simulink model "Sim1_3_simu"  (R2021a)
settings: Solver=VariableStepAuto  StartTime=0.0  StopTime=Ts*1e6  RelTol=1e-3
values from neighbouring files (symbols this model uses):
  sysd = c2d(G, Ts, 'zoh')    [Sim1_1.m]    (also in Sim1_2.m; Sim1_2_5.m; Sim1_2_CovRes_Fast.m; Sim1_2_CovRes_Slow.m)
  Ts = (2*pi)/(20*bw)    [Sim1_1.m]    (also in Sim1_2.m; Sim1_2_5.m; Sim1_2_CovRes_Fast.m; Sim1_2_CovRes_Slow.m)
undefined symbols (not defined in the file or in its folder): C
settings Model: Creator=ASUS  LastModifiedBy=ASUS

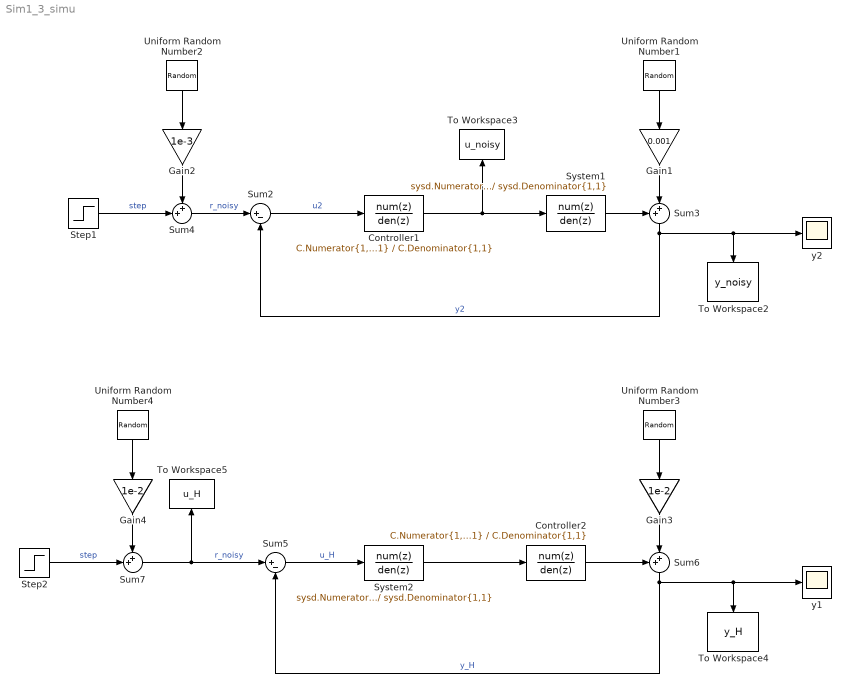
== system Sim1_3_simu ==
  Controller1 : DiscreteTransferFcn  Numerator=C.Numerator{1,1}  Denominator=C.Denominator{1,1}
  Controller2 : DiscreteTransferFcn  Numerator=C.Numerator{1,1}  Denominator=C.Denominator{1,1}
  Gain1 : Gain  Gain=0.001
  Gain2 : Gain  Gain=1e-3
  Gain3 : Gain  Gain=1e-2
  Gain4 : Gain  Gain=1e-2
  Step1 : Step  Time=0  SampleTime=0
  Step2 : Step  Time=0  SampleTime=0
  Sum2 : Sum  Inputs=|+-
  Sum{3..4,6..7} (4 alike) : Sum  Inputs=++|
  Sum5 : Sum  Inputs=|+-
  System1 : DiscreteTransferFcn  Numerator=sysd.Numerator{1,1}  Denominator=sysd.Denominator{1,1}
  System2 : DiscreteTransferFcn  Numerator=sysd.Numerator{1,1}  Denominator=sysd.Denominator{1,1}
  To Workspace2 : ToWorkspace  VariableName=y_noisy  SampleTime=-1
  To Workspace3 : ToWorkspace  VariableName=u_noisy  SampleTime=-1
  To Workspace4 : ToWorkspace  VariableName=y_H  SampleTime=-1
  To Workspace5 : ToWorkspace  VariableName=u_H  SampleTime=-1
  Uniform Random Number1 : UniformRandomNumber  SampleTime=Ts
  Uniform Random Number2 : UniformRandomNumber  Seed=1  SampleTime=Ts
  Uniform Random Number3 : UniformRandomNumber  SampleTime=Ts
  Uniform Random Number4 : UniformRandomNumber  Seed=1  SampleTime=Ts
  y1 : Scope
  y2 : Scope
  wires:
  Sum3/1 -> Sum2/2, y2/1, To Workspace2/1  "y2"
  Gain1/1 -> Sum3/2
  Uniform Random Number1/1 -> Gain1/1
  Uniform Random Number2/1 -> Gain2/1
  Gain2/1 -> Sum4/1
  Sum4/1 -> Sum2/1  "r_noisy"
  Step1/1 -> Sum4/2  "step"
  Sum2/1 -> Controller1/1  "u2"
  Sum5/1 -> System2/1  "u_H"
  Controller2/1 -> Sum6/1
  Step2/1 -> Sum7/2  "step"
  Sum7/1 -> To Workspace5/1, Sum5/1  "r_noisy"
  Gain4/1 -> Sum7/1
  Uniform Random Number4/1 -> Gain4/1
  Gain3/1 -> Sum6/2
  System2/1 -> Controller2/1
  Uniform Random Number3/1 -> Gain3/1
  Sum6/1 -> Sum5/2, y1/1, To Workspace4/1  "y_H"
  Controller1/1 -> System1/1, To Workspace3/1
  System1/1 -> Sum3/1
